simulink model "OneGFL"  (R2020a)
settings: Solver=VariableStepAuto  StartTime=0.0  StopTime=10  RelTol=1e-6
InitFcn:
  | %initAll
values from neighbouring files (symbols this model uses):
  GFLInit = GFL_init(opdata,GFL_in_gidx)    [init.m]
  Iij = -(Vm - Vc)*Y(2,1)    [init.m]
  Vm = V.*cos(del) + 1i*V.*sin(del)    [init.m]
  W0 = wB    (= 314.159265359)    [init.m]
undefined symbols (not defined in the file or in its folder): ACgirdinit
libraries: eeTransforms x3
settings Model: Creator=LinSiQi  LastModifiedBy=Qiufan_Yang
settings DebuggingCC: ArithmeticOperatorsInVariantConditions=warning
settings SFSimCC: CustomCodeUndefinedFunction=UseInterfaceOnly
settings CodeAppCC: StateflowObjectComments=on
settings SimscapeCC: SimscapeNormalizeSystem=off

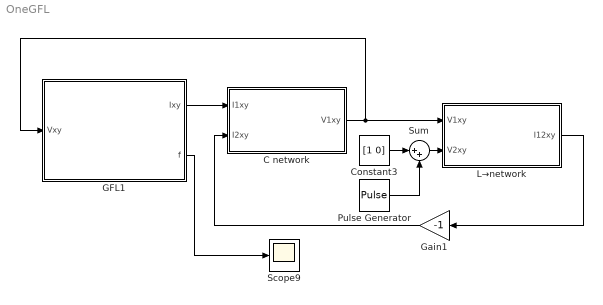
== system OneGFL ==
  C network : Subsystem  mask{C=ACgirdinit.linedata{1, 1}{1,5}/2, U1x0=real(Vm), U1y0=imag(Vm)}
  Constant3 : Constant  Value=[1 0]
  GFL1 : Subsystem  mask{Pout=-1, Qout=0, Vout=1, LG=GFLInit.LG(1), RG=GFLInit.RG(1), CF=GFLInit.CF(1), LF=GFLInit.LF(1), RF=GFLInit.RF(1), JGFL=GFLInit.J(1), DGFL=GFLInit.D(1), KPL=GFLInit.KPL(1), KIL=GFLInit.KIL(1), TFL=GFLInit.TFL(1), KPP=GFLInit.KPP(1), KIP=GFLInit.KIP(1), TPF=GFLInit.TPF(1), KPC=GFLInit.KPC(1), KIC=GFLInit.KIC(1), KVF=GFLInit.KVF(1), TVF=GFLInit.TVF(1), Pref=GFLInit.Pref(1), Qref=GFLInit.Qref(1), Vd0=GFLInit.Vd0(1), theta0=GFLInit.theta0(1), Ix0=GFLInit.Ix0(1), Iy0=GFLInit.Iy0(1), Vx0=GFLInit.Vx0(1), Vy0=GFLInit.Vy0(1), IOx0=GFLInit.IOx0(1), IOy0=GFLInit.IOy0(1), Idref0=GFLInit.Idref0(1), Iqref0=GFLInit.Iqref0(1), Ed0=GFLInit.Ed0(1), Eq0=GFLInit.Eq0(1)}
      mask init:
      | % IOxy0 = (Pout - 1i*Qout)/conj(Vout);
      | % Vxy0  = Vout + IOxy0*(RG+1i*LG);
      | % Ixy0  = IOxy0 + Vxy0*(1i*CF);
      | % Exy0  = Vxy0 + Ixy0*(RF+1i*LF);
      | % 
      | % IOx0 = real(IOxy0);
      | % IOy0 = imag(IOxy0);
      | % Vx0 = real(Vxy0);
      | % Vy0 = imag(Vxy0);
      | % Ix0 = real(Ixy0);
      | % Iy0 = imag(Ixy0);
      | % Pref = real(Vxy0*conj(IOxy0));
      | % Qref = imag(Vxy0*conj(IOxy0));
      | % Vd0  = abs(Vxy0);
      | % theta0 = angle(Vxy0);
      | % 
      | % Edq0 = abs(Exy0)*exp(1i*(angle(Exy0)-theta0));
      | % Idq0 = abs(Ixy0)*exp(1i*(angle(Ixy0)-theta0));
      | % IOdq0 = abs(IOxy0)*exp(1i*(angle(IOxy0)-theta0));
      | % 
      | % temp = Edq0 - KVF*Vd0 - Idq0*(1i*LF);
      | % Ed0 = real(temp);
      | % Eq0 = imag(temp);
      | % 
      | % Idref0 = real(Idq0);
      | % Iqref0 = imag(Idq0);
      mask DialogControl Container8 Prompt: Parameters
      mask DialogControl Container9 Prompt: Power Flow
      mask DialogControl Container6 Prompt: LCL Parameter
      mask DialogControl Container20 Prompt: Control Parameters
      mask DialogControl Container21 Prompt: Initial Parameters
  Gain1 : Gain  Gain=-1
  L→network : Subsystem  mask{L12=ACgirdinit.linedata{1, 1}{1,4}, R12=ACgirdinit.linedata{1, 1}{1,3}, Isx0=real(Iij), Isy0=imag(Iij)}
  Pulse Generator : DiscretePulseGenerator  PulseType=Time based  Period=10  PulseWidth=0.01  PhaseDelay=1
  Scope9 : Scope
  Sum : Sum  Inputs=|++
  wires:
  GFL1/1(Ixy) -> C network/1(I1xy)
  C network/1(V1xy) -> GFL1/1(Vxy), L→network/1(V1xy)
  L→network/1(I12xy) -> Gain1/1
  Gain1/1 -> C network/2(I2xy)
  GFL1/2(f) -> Scope9/1
  Constant3/1 -> Sum/1
  Sum/1 -> L→network/2(V2xy)
  Pulse Generator/1 -> Sum/2

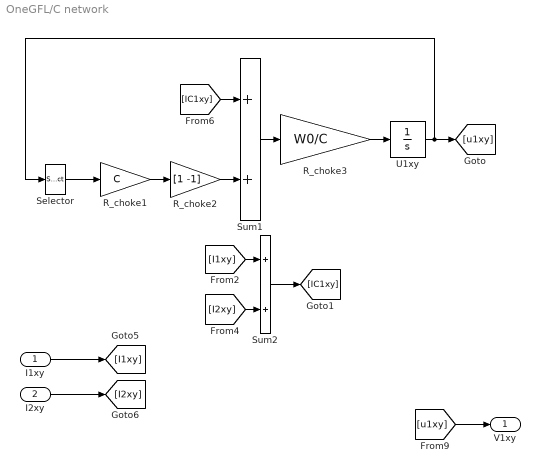
== system OneGFL/C network ==
  I1xy : Inport
  I2xy : Inport  Port=2
  R_choke1 : Gain  Gain=C  SaturateOnIntegerOverflow=on  OutDataTypeStr=Inherit: Same as input  ParamDataTypeStr=Inherit: Same as input
  R_choke2 : Gain  Gain=[1 -1]  SaturateOnIntegerOverflow=on  OutDataTypeStr=Inherit: Same as input  ParamDataTypeStr=Inherit: Same as input
  R_choke3 : Gain  Gain=W0/C  SaturateOnIntegerOverflow=on  OutDataTypeStr=Inherit: Same as input  ParamDataTypeStr=Inherit: Same as input
  Selector : Selector  InputPortWidth=2  IndexOptions=Index vector (dialog)  Indices=[2 1]  OutputSizes=1
  Sum1 : Sum  SaturateOnIntegerOverflow=on
  Sum2 : Sum  SaturateOnIntegerOverflow=on
  U1xy : Integrator  InitialCondition=[U1x0 U1y0]
  V1xy : Outport
  wires:
  I2xy/1 -> [I2xy]
  R_choke2/1 -> Sum1/2
  Sum1/1 -> R_choke3/1
  R_choke1/1 -> R_choke2/1
  I1xy/1 -> [I1xy]
  Selector/1 -> R_choke1/1
  [IC1xy] -> Sum1/1
  R_choke3/1 -> U1xy/1
  U1xy/1 -> Selector/1, [u1xy]
  [I1xy] -> Sum2/1
  Sum2/1 -> [IC1xy]
  [u1xy] -> V1xy/1
  [I2xy] -> Sum2/2

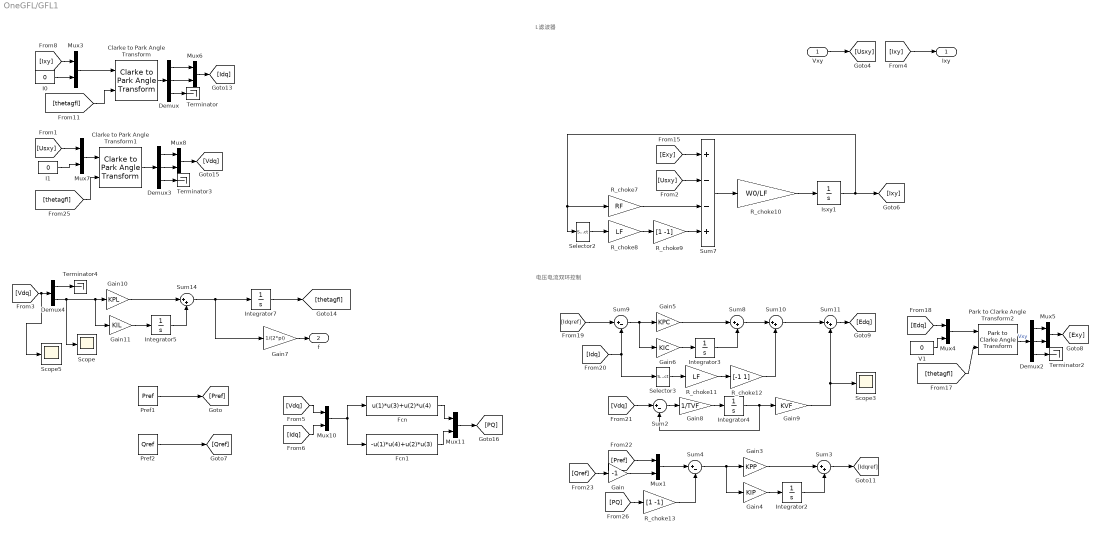
== system OneGFL/GFL1 ==
  note: 电压电流双环控制
  note: L滤波器
  Vxy : Inport
  Clarke to Park Angle Transform : eeTransforms/Clarke to Park Angle Transform  AxisAlignment=D-axis
      settings: SourceProductBaseCode=PS
  Clarke to Park Angle Transform1 : eeTransforms/Clarke to Park Angle Transform  AxisAlignment=D-axis
      settings: SourceProductBaseCode=PS
  Demux : Demux  Outputs=3
  Demux2 : Demux  Outputs=3
  Demux3 : Demux  Outputs=3
  Demux4 : Demux  Outputs=2
  Fcn : Fcn  Expr=u(1)*u(3)+u(2)*u(4)
  Fcn1 : Fcn  Expr=-u(1)*u(4)+u(2)*u(3)
  Gain : Gain  Gain=-1
  Gain10 : Gain  Gain=KPL
  Gain11 : Gain  Gain=KIL
  Gain3 : Gain  Gain=KPP
  Gain4 : Gain  Gain=KIP
  Gain5 : Gain  Gain=KPC
  Gain6 : Gain  Gain=KIC
  Gain7 : Gain  Gain=1/(2*pi)
  Gain8 : Gain  Gain=1/TVF
  Gain9 : Gain  Gain=KVF
  I0 : Constant  Value=0
  I1 : Constant  Value=0
  Integrator2 : Integrator  InitialCondition=[Idref0 Iqref0]
  Integrator3 : Integrator  InitialCondition=[Ed0 Eq0]
  Integrator4 : Integrator  InitialCondition=[Vd0 0]
  Integrator5 : Integrator
  Integrator7 : Integrator  InitialCondition=theta0
  Isxy1 : Integrator  InitialCondition=[Ix0 Iy0]
  Mux{1,3..8,10..11} (9 alike) : Mux  Inputs=2
  Park to Clarke Angle Transform2 : eeTransforms/Park to Clarke Angle Transform  AxisAlignment=D-axis
      settings: SourceProductBaseCode=PS
  Pref1 : Constant  Value=Pref
  Pref2 : Constant  Value=Qref
  R_choke10 : Gain  Gain=W0/LF  SaturateOnIntegerOverflow=on  OutDataTypeStr=Inherit: Same as input  ParamDataTypeStr=Inherit: Same as input
  R_choke11 : Gain  Gain=LF  SaturateOnIntegerOverflow=on  OutDataTypeStr=Inherit: Same as input  ParamDataTypeStr=Inherit: Same as input
  R_choke12 : Gain  Gain=[-1 1]  SaturateOnIntegerOverflow=on  OutDataTypeStr=Inherit: Same as input  ParamDataTypeStr=Inherit: Same as input
  R_choke13 : Gain  Gain=[1 -1]  SaturateOnIntegerOverflow=on  OutDataTypeStr=Inherit: Same as input  ParamDataTypeStr=Inherit: Same as input
  R_choke7 : Gain  Gain=RF  SaturateOnIntegerOverflow=on  OutDataTypeStr=Inherit: Same as input  ParamDataTypeStr=Inherit: Same as input
  R_choke8 : Gain  Gain=LF  SaturateOnIntegerOverflow=on  OutDataTypeStr=Inherit: Same as input  ParamDataTypeStr=Inherit: Same as input
  R_choke9 : Gain  Gain=[1 -1]  SaturateOnIntegerOverflow=on  OutDataTypeStr=Inherit: Same as input  ParamDataTypeStr=Inherit: Same as input
  Scope : Scope
  Scope3 : Scope
  Scope5 : Scope
  Selector2 : Selector  InputPortWidth=2  IndexOptions=Index vector (dialog)  Indices=[2 1]  OutputSizes=1
  Selector3 : Selector  InputPortWidth=2  IndexOptions=Index vector (dialog)  Indices=[2 1]  OutputSizes=1
  Sum{3,8,10..11,14} (5 alike) : Sum  Inputs=|++
  Sum2 : Sum  Inputs=|+-
  Sum4 : Sum  Inputs=|+-
  Sum7 : Sum  Inputs=+--+  SaturateOnIntegerOverflow=on
  Sum9 : Sum  Inputs=|+-
  Terminator{,2..4} (4 alike) : Terminator
  V1 : Constant  Value=0
  Ixy : Outport
  f : Outport  Port=2
  wires:
  Mux3/1 -> Clarke to Park Angle Transform/1
  I0/1 -> Mux3/2
  Demux/3 -> Terminator/1
  Demux/2 -> Mux6/2
  Demux/1 -> Mux6/1
  Clarke to Park Angle Transform/1 -> Demux/1
  Vxy/1 -> [Usxy]
  [Ixy] -> Mux3/1
  [Ixy] -> Ixy/1
  [thetagfl] -> Clarke to Park Angle Transform/2
  Gain4/1 -> Integrator2/1
  Gain3/1 -> Sum3/1
  Integrator2/1 -> Sum3/2
  Sum4/1 -> Gain4/1, Gain3/1
  Mux1/1 -> Sum4/1
  Isxy1/1 -> [Ixy], R_choke7/1, Selector2/1
  [Usxy] -> Sum7/2
  R_choke7/1 -> Sum7/3
  R_choke8/1 -> R_choke9/1
  R_choke10/1 -> Isxy1/1
  Sum7/1 -> R_choke10/1
  R_choke9/1 -> Sum7/4
  Selector2/1 -> R_choke8/1
  V1/1 -> Mux4/2
  Mux4/1 -> Park to Clarke Angle Transform2/1
  [thetagfl] -> Park to Clarke Angle Transform2/2
  Mux5/1 -> [Exy]
  Demux2/3 -> Terminator2/1
  Park to Clarke Angle Transform2/1 -> Demux2/1  "Vxy"
  Demux2/2 -> Mux5/2
  Demux2/1 -> Mux5/1
  [Idqref] -> Sum9/1
  Sum9/1 -> Gain6/1, Gain5/1
  Gain5/1 -> Sum8/1
  Gain6/1 -> Integrator3/1
  Integrator3/1 -> Sum8/2
  [Idq] -> Sum9/2, Selector3/1
  R_choke11/1 -> R_choke12/1
  Selector3/1 -> R_choke11/1
  R_choke12/1 -> Sum10/2
  Sum10/1 -> Sum11/1
  Gain9/1 -> Scope3/1, Sum11/2
  Sum11/1 -> [Edq]
  Mux6/1 -> [Idq]
  [Usxy] -> Mux7/1
  I1/1 -> Mux7/2
  Mux7/1 -> Clarke to Park Angle Transform1/1
  [thetagfl] -> Clarke to Park Angle Transform1/2
  Clarke to Park Angle Transform1/1 -> Demux3/1
  Demux3/1 -> Mux8/1
  Demux3/2 -> Mux8/2
  Mux8/1 -> [Vdq]
  Demux3/3 -> Terminator3/1
  Sum2/1 -> Gain8/1
  Gain8/1 -> Integrator4/1
  [Vdq] -> Sum2/1
  [Exy] -> Sum7/1
  Demux4/2 -> Gain11/1, Gain10/1, Scope/1
  Gain10/1 -> Sum14/1
  [Vdq] -> Scope5/1, Demux4/1
  Demux4/1 -> Terminator4/1
  Pref1/1 -> [Pref]
  Pref2/1 -> [Qref]
  [Vdq] -> Mux10/1
  [Idq] -> Mux10/2
  Mux10/1 -> Fcn1/1, Fcn/1
  Fcn/1 -> Mux11/1
  Fcn1/1 -> Mux11/2
  [Pref] -> Mux1/1
  Mux11/1 -> [PQ]
  Gain/1 -> Mux1/2
  [Qref] -> Gain/1
  [PQ] -> R_choke13/1
  R_choke13/1 -> Sum4/2
  Integrator7/1 -> [thetagfl]
  [Edq] -> Mux4/1
  Integrator4/1 -> Sum2/2, Gain9/1
  Sum8/1 -> Sum10/1
  Gain7/1 -> f/1
  Sum14/1 -> Gain7/1, Integrator7/1
  Gain11/1 -> Integrator5/1
  Integrator5/1 -> Sum14/2
  Sum3/1 -> [Idqref]

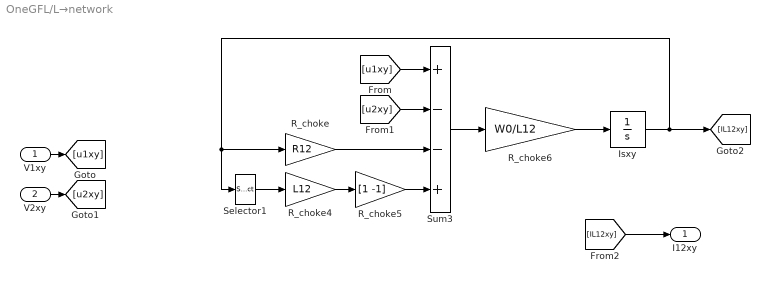
== system OneGFL/L→network ==
  V1xy : Inport
  V2xy : Inport  Port=2
  Isxy : Integrator  InitialCondition=[Isx0 Isy0]
  R_choke : Gain  Gain=R12  SaturateOnIntegerOverflow=on  OutDataTypeStr=Inherit: Same as input  ParamDataTypeStr=Inherit: Same as input
  R_choke4 : Gain  Gain=L12  SaturateOnIntegerOverflow=on  OutDataTypeStr=Inherit: Same as input  ParamDataTypeStr=Inherit: Same as input
  R_choke5 : Gain  Gain=[1 -1]  SaturateOnIntegerOverflow=on  OutDataTypeStr=Inherit: Same as input  ParamDataTypeStr=Inherit: Same as input
  R_choke6 : Gain  Gain=W0/L12  SaturateOnIntegerOverflow=on  OutDataTypeStr=Inherit: Same as input  ParamDataTypeStr=Inherit: Same as input
  Selector1 : Selector  InputPortWidth=2  IndexOptions=Index vector (dialog)  Indices=[2 1]  OutputSizes=1
  Sum3 : Sum  Inputs=+--+  SaturateOnIntegerOverflow=on
  I12xy : Outport
  wires:
  R_choke5/1 -> Sum3/4
  [u2xy] -> Sum3/2
  R_choke4/1 -> R_choke5/1
  Sum3/1 -> R_choke6/1
  Selector1/1 -> R_choke4/1
  R_choke6/1 -> Isxy/1
  [u1xy] -> Sum3/1
  R_choke/1 -> Sum3/3
  Isxy/1 -> [IL12xy], R_choke/1, Selector1/1
  V1xy/1 -> [u1xy]
  V2xy/1 -> [u2xy]
  [IL12xy] -> I12xy/1
